simulink model "tempDAQ"  (R2022b)
settings: Solver=FixedStepAuto  StartTime=0.0  StopTime=60  RelTol=1e-3  EnableMultiTasking=on
libraries: arduinolib x1, arduinomotorcarrierlib x1
settings Model: ExtModeTrigDuration=2  Creator=EMD LAB  LastModifiedBy=EMD LAB
settings OptimizationCC: EnhancedBackFolding=on  PassReuseOutputArgsAs=Individual arguments  ZeroExternalMemoryAtStartup=off  ZeroInternalMemoryAtStartup=off  MaxStackSize=64  OptimizeBlockOrder=speed  DifferentSizesBufferReuse=on  OptimizationCustomize=off  EfficientTunableParamExpr=on
settings DebuggingCC: ParameterTunabilityLossMsg=error
settings HardwareCC: ProdBitPerInt=16  ProdBitPerPointer=16  ProdBitPerSizeT=16  ProdBitPerPtrDiffT=16  ProdLargestAtomicFloat=None  ProdWordSize=8  ProdHWDeviceType=Atmel->AVR
settings SFSimCC: MATLABDynamicMemAlloc=off
settings RTWCC: Description=Embedded Coder  SystemTargetFile=ert.tlc  HardwareBoard=Arduino Mega 2560  TLCOptions=-aInlineSetEventsForThisBaseRateFcn=TLC_FALSE -aSuppressMultiTaskScheduler=TLC_FALSE -aRateBasedStepFcn=1  TemplateMakefile=ert_default_tmf  Toolchain=Arduino AVR  BuildConfiguration=Faster Runs
settings CodeAppCC: ForceParamTrailComments=on  IgnoreCustomStorageClasses=off  OperatorAnnotations=on  SimulinkDataObjDesc=on  SFDataObjDesc=on  InsertBlockDesc=on
settings ERTTargetCC: SupportContinuousTime=on  SupportVariableSizeSignals=on  ExtModeTransport=3  ExtModeStaticAlloc=on  ExtModeAutomaticAllocSize=off  ExtModeStaticAllocSize=2048  ExtModeMexFile=ext_xcp  ExtModeIntrfLevel=Level2 - Open

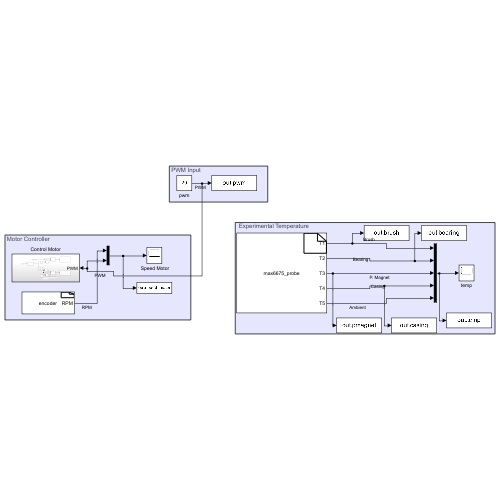
[thumbnail: Simulink's stored preview of the top-level diagram]
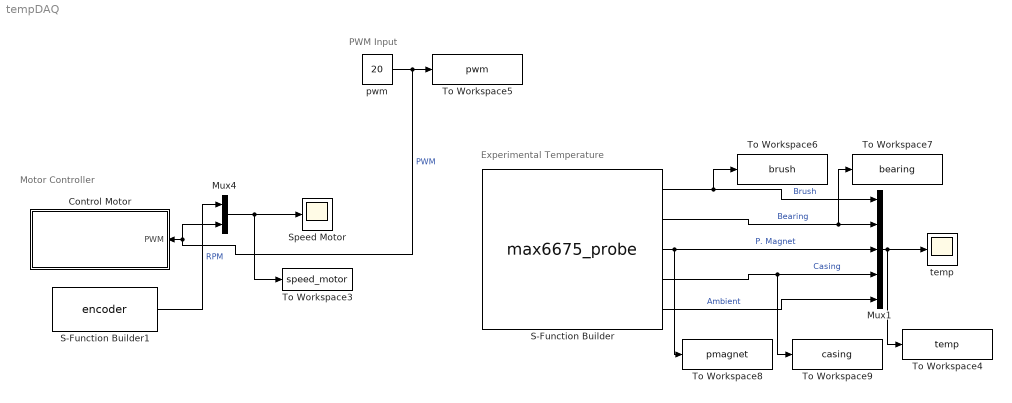
== system tempDAQ ==
  note: PWM Input
  note: Experimental Temperature
  note: Motor Controller
  " Speed Motor" : Scope
  Control Motor : Subsystem
  Mux1 : Mux  Inputs=5
  Mux4 : Mux  Inputs=2
  S-Function Builder : S-Function  FunctionName=max6675_probe  SFunctionModules=max6675_probe_wrapper.cpp  SFunctionDeploymentMode=off  EnableBusSupport=off  mask(S-Function Builder){}
      mask help: Simulink:masks:SFunctionBuilder_MD
      mask init:
      | val = [[.9  0.75 0.75 1 1 .9 .9 1]',[1 1 0.75 0.75 .9 .9 1 .9]'];try , sys = get_param(gcb,'SfunBuilderFcnName');if isempty(sys), sys = get_param(gcb,'FunctionName'); end,catch, sys = get_param(gcb,'FunctionName'); end
      settings: CopyFcn=set_param(gcbh,'LinkStatus','none')  OpenFcn=sfunctionwizard(gcbh)
      mask Display:
      | plot(val(:,1),val(:,2))
      | disp(sys)
      | port_label('output',1,'T1')
      | port_label('output',2,'T2')
      | port_label('output',3,'T3')
      | port_label('output',4,'T4')
      | port_label('output',5,'T5')
  S-Function Builder1 : S-Function  FunctionName=encoder  SFunctionModules=encoder_wrapper.cpp  SFunctionDeploymentMode=off  EnableBusSupport=off  mask(S-Function Builder){}
      mask help: Simulink:masks:SFunctionBuilder_MD
      mask init: same as tempDAQ/S-Function Builder
      settings: CopyFcn=set_param(gcbh,'LinkStatus','none')  OpenFcn=sfunctionwizard(gcbh)
      mask Display:
      | plot(val(:,1),val(:,2))
      | disp(sys)
      | port_label('output',1,'RPM')
  To Workspace3 : ToWorkspace  VariableName=speed_motor  SaveFormat=Structure With Time  SampleTime=-1
  To Workspace4 : ToWorkspace  VariableName=temp  SaveFormat=Structure With Time  SampleTime=-1
  To Workspace5 : ToWorkspace  VariableName=pwm  SaveFormat=Structure With Time  SampleTime=-1
  To Workspace6 : ToWorkspace  VariableName=brush  SaveFormat=Structure With Time  SampleTime=-1
  To Workspace7 : ToWorkspace  VariableName=bearing  SaveFormat=Structure With Time  SampleTime=-1
  To Workspace8 : ToWorkspace  VariableName=pmagnet  SaveFormat=Structure With Time  SampleTime=-1
  To Workspace9 : ToWorkspace  VariableName=casing  SaveFormat=Structure With Time  SampleTime=-1
  pwm : Constant  Value=20  VectorParams1D=off
  temp : Scope
  wires:
  S-Function Builder1/1 -> Mux4/1  "RPM"
  S-Function Builder/5 -> Mux1/5  "Ambient"
  pwm/1 -> Mux4/2, Control Motor/1(PWM), To Workspace5/1  "PWM"
  S-Function Builder/4 -> Mux1/4, To Workspace9/1  "Casing"
  Mux1/1 -> temp/1, To Workspace4/1
  Mux4/1 -> " Speed Motor"/1, To Workspace3/1
  S-Function Builder/1 -> Mux1/1, To Workspace6/1  "Brush"
  S-Function Builder/2 -> Mux1/2, To Workspace7/1  "Bearing"
  S-Function Builder/3 -> To Workspace8/1, Mux1/3  "P. Magnet"

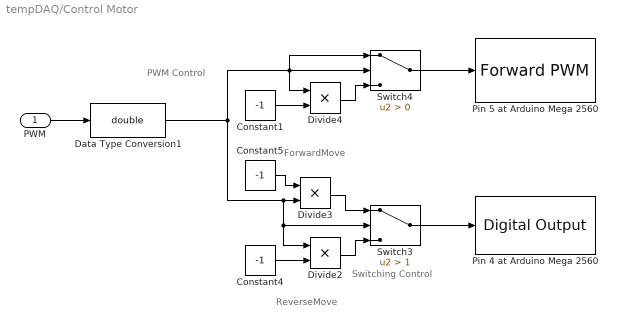
== system tempDAQ/Control Motor ==
  note: PWM Control
  note: ReverseMove
  note: ForwardMove
  note: Switching Control
  PWM : Inport
  Constant1 : Constant  Value=-1
  Constant4 : Constant  Value=-1
  Constant5 : Constant  Value=-1
  Data Type Conversion1 : DataTypeConversion  OutDataTypeStr=double  SaturateOnIntegerOverflow=off  RndMeth=Floor
  Divide2 : Product  Inputs=**
  Divide3 : Product  Inputs=**
  Divide4 : Product  Inputs=**
  Pin 4 at Arduino Mega 2560 : arduinolib/Digital Output  pinNumber=4  Direction=output  blockPlatform=arduino
  Pin 5 at Arduino Mega 2560 : arduinomotorcarrierlib/M3 M4 DC Motors/Forward PWM  pinNumber=5  EnableInputFrequency=off  InitialFrequency=2000  InitialDutyCycle=0  NotificationType=None  timerPeriod=0  timerPrescaler=0  frequencyType=Default  desiredFrequency=490.2  blockPlatform=arduino
  Switch3 : Switch  Criteria=u2 > Threshold  Threshold=1  SaturateOnIntegerOverflow=off  InputSameDT=off
  Switch4 : Switch  Criteria=u2 > Threshold  SaturateOnIntegerOverflow=off  InputSameDT=off
  wires:
  PWM/1 -> Data Type Conversion1/1
  Divide2/1 -> Switch3/3
  Constant4/1 -> Divide2/2
  Divide3/1 -> Switch3/1
  Data Type Conversion1/1 -> Switch3/2, Divide2/1, Divide3/2, Switch4/1, Switch4/2, Divide4/1
  Constant5/1 -> Divide3/1
  Switch3/1 -> Pin 4 at Arduino Mega 2560/1
  Constant1/1 -> Divide4/2
  Divide4/1 -> Switch4/3
  Switch4/1 -> Pin 5 at Arduino Mega 2560/1
